simulink model "SysConfStateMachTest"  (R2012b)
settings: Solver=ode1  StartTime=0.0  StopTime=Inf  FixedStep=Tsample_simulink  RelTol=1e-3
PostLoadFcn:
  | , if any(exist('dsrtsu_mdlpostloadfcn', 'file') == [2, 3, 6]), try dsrtsu_mdlpostloadfcn('Execute', bdroot); catch fprintf('Error in PostLoadFcn (dsrtsu_mdlpostloadfcn) for model "%s":\n %s\n', bdroot, lasterr); end, end,
values from neighbouring files (symbols this model uses):
  Tsample_simulink = Ts/10    (= 2e-05)    [load_system_parameters.m]
libraries: simulink_extras x2
(part 2 of 9)

== matlab function SysConfStateMachTest/MATLAB Function1 ==
  data: profile_on input; command_output output; simulation_time input
function command_output = generate_profile(profile_on, simulation_time)

persistent profile_on_condition index last_time period command profile;

if isempty(profile_on_condition)
    profile_on_condition = 5;
end
if isempty(index)
    index = 0;
end
if isempty(last_time)
    last_time = simulation_time;
end
if isempty(period)
    period = 1/10;
end
if isempty(command)
    command = 0;
end
if isempty(profile)
